simulink model "pose_contour"  (R2023a)
settings: Solver=VariableStepAuto  StartTime=0.0  StopTime=3  MaxStep=1e-4  RelTol=1e-3
values from neighbouring files (symbols this model uses):
  a_max = 1    [init_simulink.m]
  err_pose = 0.005    [init_simulink.m]
  i = 262    [init_simulink.m]
  J = 3.29e-3    (= 0.00329)    [init_simulink.m]
  k_curr = 1    [init_simulink.m]
  k_pow = 10    [init_simulink.m]
  ki_curr = (r_coeff * R) / (k_curr * k_pow)    (= 123.75)    [init_simulink.m]
  km = 0.98    [init_simulink.m]
  kp_curr = ki_curr * T_e    (= 0.8415)    [init_simulink.m]
  kw = 0.98    [init_simulink.m]
  Q = nominal_torque * 0.7    (= 3.29)    [init_simulink.m]
  R = 0.99    [init_simulink.m]
  t_accel = 0.8    [init_simulink.m]
  t_braking = 0.8    [init_simulink.m]
  t_const_rate = 1    [init_simulink.m]
  T_e = 0.0068    [init_simulink.m]
  T_pow = 0.0004    [init_simulink.m]
libraries: simulink x4
settings Model: Creator=k.balkunov  LastModifiedBy=k.balkunov

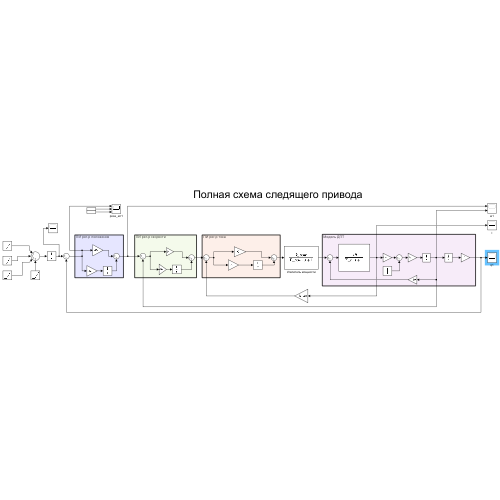
[thumbnail: Simulink's stored preview of the top-level diagram]
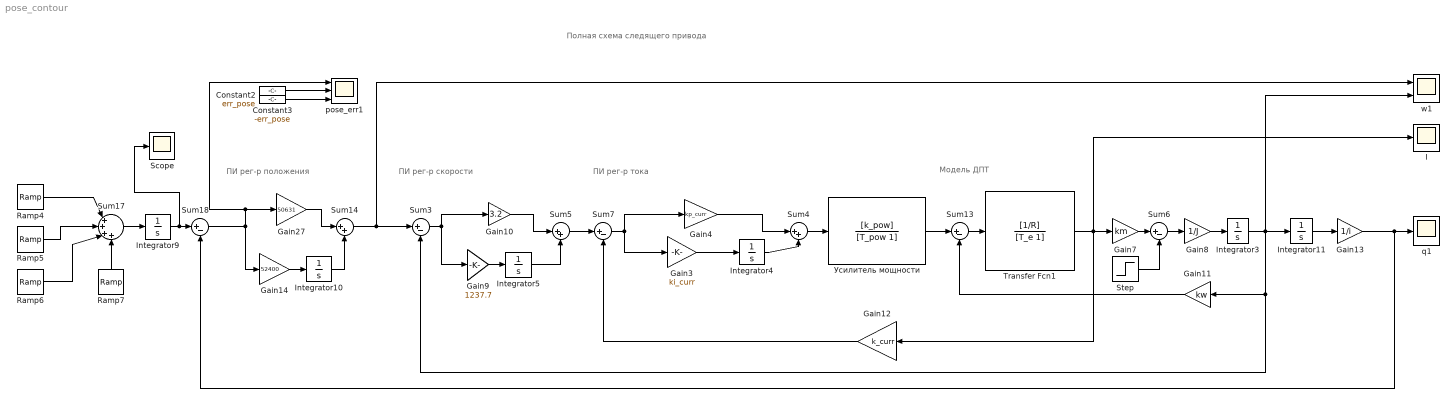
== system pose_contour ==
  note: Полная схема следящего привода
  note: ПИ рег-р положения
  note: ПИ рег-р тока
  note: ПИ рег-р скорости
  note: Модель ДПТ
  Constant2 : Constant  Value=err_pose
  Constant3 : Constant  Value=-err_pose
  Gain10 : Gain  Gain=3.2
  Gain11 : Gain  Gain=kw
  Gain12 : Gain  Gain=k_curr
  Gain13 : Gain  Gain=1/i
  Gain14 : Gain  Gain=52400
  Gain27 : Gain  Gain=50631
  Gain3 : Gain  Gain=ki_curr
  Gain4 : Gain  Gain=kp_curr
  Gain7 : Gain  Gain=km
  Gain8 : Gain  Gain=1/J
  Gain9 : Gain  Gain=1237.7
  I : Scope
  Integrator{3..5,9..11} (6 alike) : Integrator
  Ramp4 : simulink/Sources/Ramp  slope=a_max  start=0  InitialOutput=0
  Ramp5 : simulink/Sources/Ramp  slope=-a_max  start=t_accel  InitialOutput=0
  Ramp6 : simulink/Sources/Ramp  slope=-a_max  start=t_accel + t_const_rate  InitialOutput=0
  Ramp7 : simulink/Sources/Ramp  slope=a_max  start=t_accel + t_const_rate + t_braking  InitialOutput=0
  Scope : Scope
  Step : Step  After=Q  SampleTime=0
  Sum{3,6..7,13,18} (5 alike) : Sum  Inputs=|+-
  Sum14 : Sum  Inputs=|++
  Sum17 : Sum  Inputs=|++++
  Sum4 : Sum  Inputs=|++
  Sum5 : Sum  Inputs=|++
  Transfer Fcn1 : TransferFcn  Numerator=[1/R]  Denominator=[T_e 1]
  pose_err1 : Scope  NumInputPorts=3
  q1 : Scope
  w1 : Scope  NumInputPorts=2
  Усилитель мощности : TransferFcn  Numerator=[k_pow]  Denominator=[T_pow 1]
  wires:
  Gain9/1 -> Integrator5/1
  Transfer Fcn1/1 -> Gain12/1, I/1, Gain7/1
  Sum7/1 -> Gain4/1, Gain3/1
  Sum13/1 -> Transfer Fcn1/1
  Sum4/1 -> Усилитель мощности/1
  Gain8/1 -> Integrator3/1
  Gain3/1 -> Integrator4/1
  Усилитель мощности/1 -> Sum13/1
  Gain4/1 -> Sum4/1
  Integrator4/1 -> Sum4/2
  Sum5/1 -> Sum7/1
  Gain11/1 -> Sum13/2
  Gain10/1 -> Sum5/1
  Sum3/1 -> Gain9/1, Gain10/1
  Gain12/1 -> Sum7/2
  Sum14/1 -> w1/1, Sum3/1
  Integrator5/1 -> Sum5/2
  Integrator3/1 -> Sum3/2, Gain11/1, Integrator11/1, w1/2
  Constant3/1 -> pose_err1/2
  Integrator9/1 -> Scope/1, Sum18/1
  Integrator11/1 -> Gain13/1
  Sum17/1 -> Integrator9/1
  Gain13/1 -> Sum18/2, q1/1
  Integrator10/1 -> Sum14/2
  Gain27/1 -> Sum14/1
  Sum18/1 -> Gain14/1, pose_err1/1, Gain27/1
  Gain14/1 -> Integrator10/1
  Ramp6/1 -> Sum17/3
  Ramp5/1 -> Sum17/2
  Ramp7/1 -> Sum17/4
  Ramp4/1 -> Sum17/1
  Constant2/1 -> pose_err1/3
  Gain7/1 -> Sum6/1
  Sum6/1 -> Gain8/1
  Step/1 -> Sum6/2
